simulink model "Bebop_sim"  (R2018a)
settings: Solver=VariableStepAuto  StartTime=0.0  StopTime=10.0  RelTol=1e-3
values from neighbouring files (symbols this model uses):
  I = [1 0 0 ... (first row only)    [Bebop_sim_init.m]
  mass = 2    [Bebop_sim_init.m]
  max_rot_Z = (90)*pi/180    (= 1.57079632679)    [Bebop_sim_init.m]
  max_theta_X = (40)*pi/180    (= 0.698131700798)    [Bebop_sim_init.m]
  max_theta_Y = (40)*pi/180    (= 0.698131700798)    [Bebop_sim_init.m]
  max_v_Z = 1.5    [Bebop_sim_init.m]
libraries: aerolibactuator x2, simulink x2, shared6dof x1, aerolibanimutils x1
settings Model: EnablePacing=on  Creator=derek  LastModifiedBy=derek

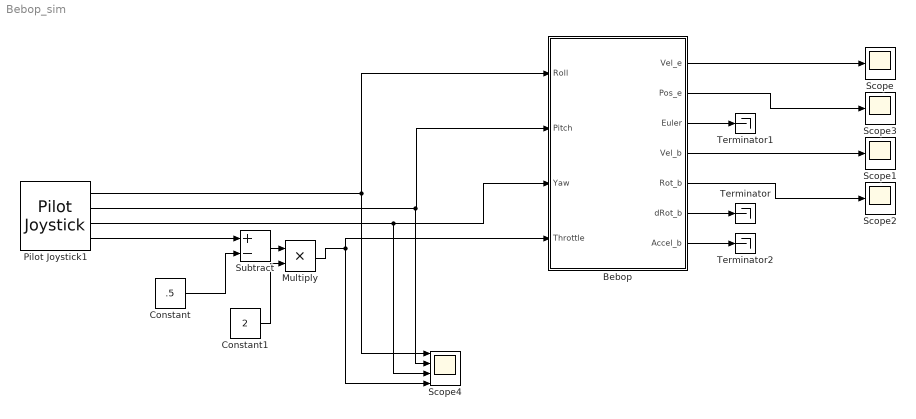
== system Bebop_sim ==
  Bebop : Subsystem
  Constant : Constant  Value=.5
  Constant1 : Constant  Value=2
  Multiply : Product
  Pilot Joystick1 : aerolibanimutils/Pilot Joystick  JoystickID=Joystick1  OutputConfiguration=FourAxis  SampleTime=1/30
  Scope{,1..3} (4 alike) : Scope
  Scope4 : Scope  NumInputPorts=4
  Subtract : Sum  Inputs=+-
  Terminator : Terminator
  Terminator1 : Terminator
  Terminator2 : Terminator
  wires:
  Pilot Joystick1/1 -> Bebop/1(Roll), Scope4/1
  Pilot Joystick1/2 -> Scope4/2, Bebop/2(Pitch)
  Pilot Joystick1/3 -> Scope4/3, Bebop/3(Yaw)
  Multiply/1 -> Bebop/4(Throttle), Scope4/4
  Bebop/1(Vel_e) -> Scope/1
  Bebop/4(Vel_b) -> Scope1/1
  Bebop/5(Rot_b) -> Scope2/1
  Bebop/2(Pos_e) -> Scope3/1
  Bebop/7(Accel_b) -> Terminator2/1
  Bebop/6(dRot_b) -> Terminator/1
  Bebop/3(Euler) -> Terminator1/1
  Pilot Joystick1/4 -> Subtract/1
  Subtract/1 -> Multiply/1
  Constant/1 -> Subtract/2
  Constant1/1 -> Multiply/2

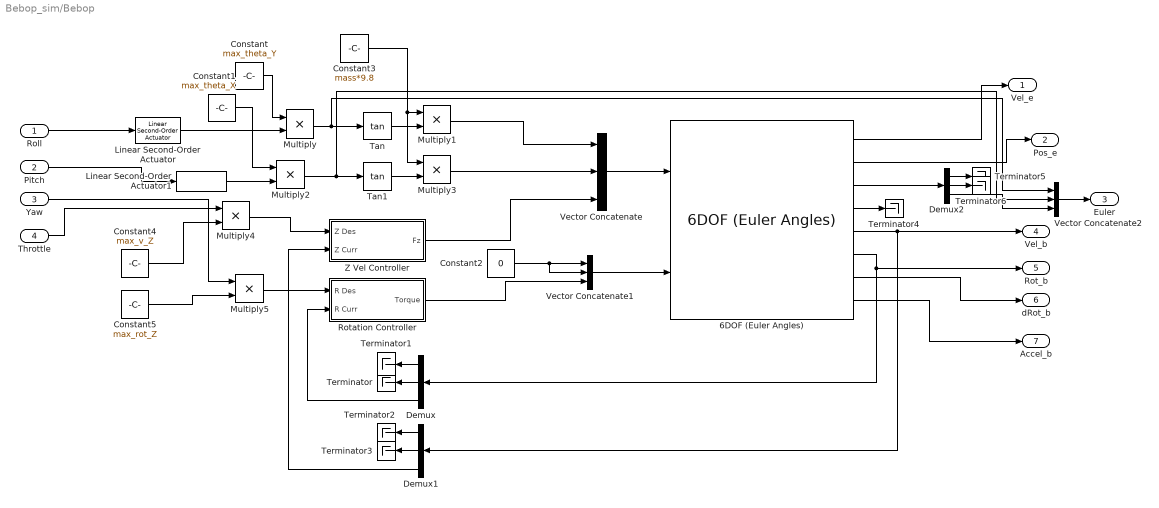
== system Bebop_sim/Bebop ==
  Roll : Inport
  Pitch : Inport  Port=2
  Yaw : Inport  Port=3
  Throttle : Inport  Port=4
  6DOF (Euler Angles) : shared6dof/6DOF (Euler Angles)  units=Metric (MKS)  mtype=Fixed  rep=Euler Angles  xme_0=Initial_pos  Vm_0=Initial_vel_b  eul_0=[0 0 0]  pm_0=[0 0 0]  mass_0=mass  mass_e=0.5  mass_f=2.0  inertia=I  inertia_e=eye(3)  inertia_f=2*eye(3)  k_quat=1.0  vre_flag=on  abi_flag=off  aMode=0
      settings: SourceProductBaseCode=AE
  Constant : Constant  Value=max_theta_Y
  Constant1 : Constant  Value=max_theta_X
  Constant2 : Constant  Value=0
  Constant3 : Constant  Value=mass*9.8
  Constant4 : Constant  Value=max_v_Z
  Constant5 : Constant  Value=max_rot_Z
  Demux : Demux  Outputs=3
  Demux1 : Demux  Outputs=3
  Demux2 : Demux  Outputs=3
  Linear Second-Order Actuator : aerolibactuator/Linear Second-Order Actuator  wn_fin=20  z_fin=1  fin_act_0=0  fin_act_vel=0
      settings: SourceProductName=Aerospace Blockset  SourceProductBaseCode=AE
  Linear Second-Order Actuator1 : aerolibactuator/Linear Second-Order Actuator  wn_fin=20  z_fin=1  fin_act_0=0  fin_act_vel=0
      settings: SourceProductName=Aerospace Blockset  SourceProductBaseCode=AE
  Multiply{,1..5} (6 alike) : Product
  Rotation Controller : Subsystem
  Tan : Trigonometry  Operator=tan
  Tan1 : Trigonometry  Operator=tan
  Terminator{,1..6} (7 alike) : Terminator
  Vector Concatenate : Concatenate  NumInputs=3
  Vector Concatenate1 : Concatenate  NumInputs=3
  Vector Concatenate2 : Concatenate  NumInputs=3
  Z Vel Controller : Subsystem
  Vel_e : Outport
  Pos_e : Outport  Port=2
  Euler : Outport  Port=3
  Vel_b : Outport  Port=4
  Rot_b : Outport  Port=5
  dRot_b : Outport  Port=6
  Accel_b : Outport  Port=7
  wires:
  Demux1/2 -> Terminator3/1
  Demux/2 -> Terminator/1
  Demux/1 -> Terminator1/1
  Constant4/1 -> Multiply4/2
  Yaw/1 -> Multiply5/1
  Multiply5/1 -> Rotation Controller/1(R Des)
  Vector Concatenate1/1 -> 6DOF (Euler Angles)/2
  Multiply4/1 -> Z Vel Controller/1(Z Des)
  Throttle/1 -> Multiply4/1
  Constant5/1 -> Multiply5/2
  Constant/1 -> Multiply/1
  Demux1/1 -> Terminator2/1
  Pitch/1 -> Linear Second-Order Actuator1/1
  Multiply3/1 -> Vector Concatenate/2
  Tan/1 -> Multiply1/2
  Constant2/1 -> Vector Concatenate1/2, Vector Concatenate1/1
  Multiply2/1 -> Vector Concatenate2/2, Tan1/1
  Tan1/1 -> Multiply3/2
  Constant1/1 -> Multiply2/1
  Constant3/1 -> Multiply1/1, Multiply3/1
  Rotation Controller/1(Torque) -> Vector Concatenate1/3
  Z Vel Controller/1(Fz) -> Vector Concatenate/3
  Demux1/3 -> Z Vel Controller/2(Z Curr)
  Multiply/1 -> Vector Concatenate2/1, Tan/1
  Demux/3 -> Rotation Controller/2(R Curr)
  Multiply1/1 -> Vector Concatenate/1
  Roll/1 -> Linear Second-Order Actuator/1
  6DOF (Euler Angles)/5 -> Demux1/1, Vel_b/1
  Vector Concatenate/1 -> 6DOF (Euler Angles)/1
  6DOF (Euler Angles)/6 -> Rot_b/1, Demux/1
  6DOF (Euler Angles)/2 -> Pos_e/1
  6DOF (Euler Angles)/1 -> Vel_e/1
  6DOF (Euler Angles)/7 -> dRot_b/1
  6DOF (Euler Angles)/8 -> Accel_b/1
  6DOF (Euler Angles)/4 -> Terminator4/1
  Linear Second-Order Actuator/1 -> Multiply/2
  Linear Second-Order Actuator1/1 -> Multiply2/2
  6DOF (Euler Angles)/3 -> Demux2/1
  Vector Concatenate2/1 -> Euler/1
  Demux2/3 -> Vector Concatenate2/3
  Demux2/2 -> Terminator6/1
  Demux2/1 -> Terminator5/1

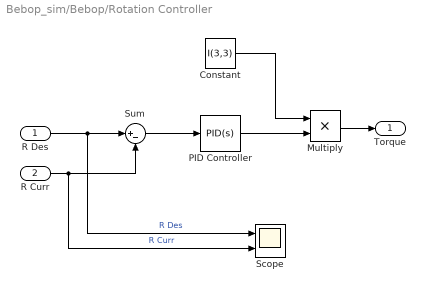
== system Bebop_sim/Bebop/Rotation Controller ==
  R Des : Inport
  R Curr : Inport  Port=2
  Constant : Constant  Value=I(3,3)
  Multiply : Product
  PID Controller : simulink/Continuous/PID Controller  Controller=PID  TimeDomain=Continuous-time  SampleTime=-1  IntegratorMethod=Forward Euler  FilterMethod=Forward Euler  Form=Parallel  UseFilter=on  ControllerParametersSource=internal  P=10  I=.3  D=.1  N=100  InitialConditionSource=internal  InitialConditionForIntegrator=0  InitialConditionForFilter=0  ExternalReset=none  LimitOutput=off  UpperSaturationLimit=inf  LowerSaturationLimit=-inf  LinearizeAsGain=on  AntiWindupMode=none  Kb=1  TrackingMode=off  Kt=1  PParamMin=[]  PParamMax=[]  IParamMin=[]  IParamMax=[]  DParamMin=[]  DParamMax=[]  NParamMin=[]  NParamMax=[]  KbParamMin=[]  KbParamMax=[]  KtParamMin=[]  KtParamMax=[]  POutMin=[]  POutMax=[]  IOutMin=[]  IOutMax=[]  DOutMin=[]  DOutMax=[]  NOutMin=[]  NOutMax=[]  KbOutMin=[]  KbOutMax=[]  KtOutMin=[]  KtOutMax=[]  IntegratorOutMin=[]  IntegratorOutMax=[]  FilterOutMin=[]  FilterOutMax=[]  SumOutMin=[]  SumOutMax=[]  SumI1OutMin=[]  SumI1OutMax=[]  SumI2OutMin=[]  SumI2OutMax=[]  SumI3OutMin=[]  SumI3OutMax=[]  SumDOutMin=[]  SumDOutMax=[]  SaturationOutMin=[]  SaturationOutMax=[]  IntegratorContinuousStateAttributes=''  IntegratorStateMustResolveToSignalObject=off  IntegratorRTWStateStorageClass=Auto  FilterContinuousStateAttributes=''  FilterStateMustResolveToSignalObject=off  FilterRTWStateStorageClass=Auto  DifferentiatorICPrevScaledInput=0  DifferentiatorOutMin=[]  DifferentiatorOutMax=[]  FilterDiffOutCoefMin=[]  FilterDiffOutCoefMax=[]  SumDenOutMin=[]  SumDenOutMax=[]  SumNumOutMin=[]  SumNumOutMax=[]  ReciprocalOutMin=[]  ReciprocalOutMax=[]  DivideOutMin=[]  DivideOutMax=[]  TunerSelectOption=Transfer Function Based (PID Tuner App)
  Scope : Scope  NumInputPorts=2
  Sum : Sum  Inputs=|+-
  Torque : Outport
  wires:
  R Des/1 -> Scope/1, Sum/1  "R Des"
  PID Controller/1 -> Multiply/2
  Sum/1 -> PID Controller/1
  Multiply/1 -> Torque/1
  R Curr/1 -> Scope/2, Sum/2  "R Curr"
  Constant/1 -> Multiply/1

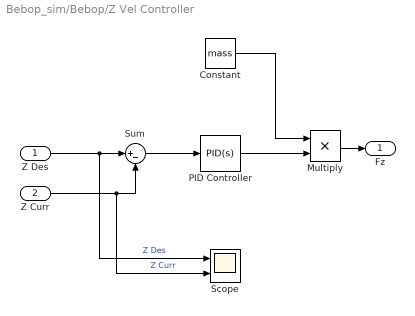
== system Bebop_sim/Bebop/Z Vel Controller ==
  Z Des : Inport
  Z Curr : Inport  Port=2
  Constant : Constant  Value=mass
  Multiply : Product
  PID Controller : simulink/Continuous/PID Controller  Controller=PID  TimeDomain=Continuous-time  SampleTime=-1  IntegratorMethod=Forward Euler  FilterMethod=Forward Euler  Form=Parallel  UseFilter=on  ControllerParametersSource=internal  P=5  I=.15  D=.1  N=100  InitialConditionSource=internal  InitialConditionForIntegrator=0  InitialConditionForFilter=0  ExternalReset=none  LimitOutput=off  UpperSaturationLimit=inf  LowerSaturationLimit=-inf  LinearizeAsGain=on  AntiWindupMode=none  Kb=1  TrackingMode=off  Kt=1  PParamMin=[]  PParamMax=[]  IParamMin=[]  IParamMax=[]  DParamMin=[]  DParamMax=[]  NParamMin=[]  NParamMax=[]  KbParamMin=[]  KbParamMax=[]  KtParamMin=[]  KtParamMax=[]  POutMin=[]  POutMax=[]  IOutMin=[]  IOutMax=[]  DOutMin=[]  DOutMax=[]  NOutMin=[]  NOutMax=[]  KbOutMin=[]  KbOutMax=[]  KtOutMin=[]  KtOutMax=[]  IntegratorOutMin=[]  IntegratorOutMax=[]  FilterOutMin=[]  FilterOutMax=[]  SumOutMin=[]  SumOutMax=[]  SumI1OutMin=[]  SumI1OutMax=[]  SumI2OutMin=[]  SumI2OutMax=[]  SumI3OutMin=[]  SumI3OutMax=[]  SumDOutMin=[]  SumDOutMax=[]  SaturationOutMin=[]  SaturationOutMax=[]  IntegratorContinuousStateAttributes=''  IntegratorStateMustResolveToSignalObject=off  IntegratorRTWStateStorageClass=Auto  FilterContinuousStateAttributes=''  FilterStateMustResolveToSignalObject=off  FilterRTWStateStorageClass=Auto  DifferentiatorICPrevScaledInput=0  DifferentiatorOutMin=[]  DifferentiatorOutMax=[]  FilterDiffOutCoefMin=[]  FilterDiffOutCoefMax=[]  SumDenOutMin=[]  SumDenOutMax=[]  SumNumOutMin=[]  SumNumOutMax=[]  ReciprocalOutMin=[]  ReciprocalOutMax=[]  DivideOutMin=[]  DivideOutMax=[]  TunerSelectOption=Transfer Function Based (PID Tuner App)
  Scope : Scope  NumInputPorts=2
  Sum : Sum  Inputs=|+-
  Fz : Outport
  wires:
  Z Des/1 -> Scope/1, Sum/1  "Z Des"
  Z Curr/1 -> Scope/2, Sum/2  "Z Curr"
  Sum/1 -> PID Controller/1
  Multiply/1 -> Fz/1
  PID Controller/1 -> Multiply/2
  Constant/1 -> Multiply/1
